simulink model "gyroscope_test"  (R2019a)
settings: Solver=FixedStepAuto  StartTime=0.0  StopTime=30  FixedStep=0.001  RelTol=1e-3
undefined symbols (not defined in the file): gyro_noise
libraries: simulink x6, simulink_extras x5, aerolibnav x2
settings Model: Creator=asmialek  LastModifiedBy=asmialek

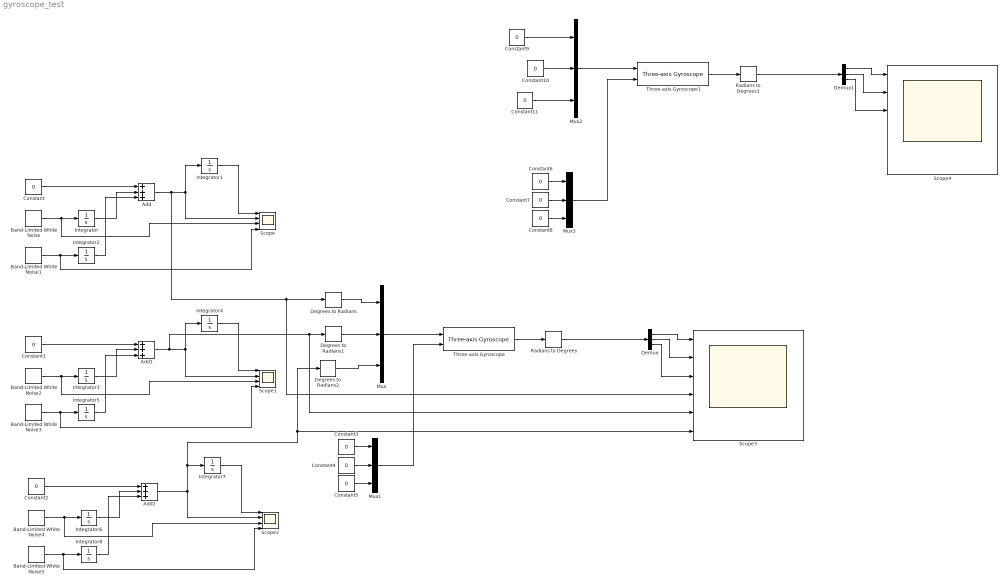
== system gyroscope_test ==
  Add : Sum  Inputs=+++
  Add1 : Sum  Inputs=+++
  Add2 : Sum  Inputs=+++
  Band-Limited White Noise : simulink/Sources/Band-Limited White Noise  Cov=0.002  Ts=10  seed=[233341]
  Band-Limited White Noise1 : simulink/Sources/Band-Limited White Noise  Cov=0.00001  Ts=1  seed=[23341]
  Band-Limited White Noise2 : simulink/Sources/Band-Limited White Noise  Cov=0.002  Ts=10  seed=[233341]
  Band-Limited White Noise3 : simulink/Sources/Band-Limited White Noise  Cov=0.00001  Ts=1  seed=[23341]
  Band-Limited White Noise4 : simulink/Sources/Band-Limited White Noise  Cov=0.002  Ts=10  seed=[233341]
  Band-Limited White Noise5 : simulink/Sources/Band-Limited White Noise  Cov=0.00001  Ts=1  seed=[23341]
  Constant{,1..11} (12 alike) : Constant  Value=0
  Degrees to Radians : simulink_extras/Transformations/Degrees to Radians
  Degrees to Radians1 : simulink_extras/Transformations/Degrees to Radians
  Degrees to Radians2 : simulink_extras/Transformations/Degrees to Radians
  Demux : Demux  Outputs=3
  Demux1 : Demux  Outputs=3
  Integrator{,1..8} (9 alike) : Integrator
  Mux{,1..3} (4 alike) : Mux  Inputs=3
  Radians to Degrees : simulink_extras/Transformations/Radians to Degrees
  Radians to Degrees1 : simulink_extras/Transformations/Radians to Degrees
  Scope : Scope  NumInputPorts=4
  Scope1 : Scope  NumInputPorts=4
  Scope2 : Scope  NumInputPorts=4
  Scope3 : Scope  NumInputPorts=6
  Scope4 : Scope  NumInputPorts=6
  Three-axis Gyroscope : aerolibnav/Three-axis Gyroscope  dtype_g=on  w_g=1  z_g=0  g_sf_cc=[1 0 0; 0 1 0; 0 0 1]  g_bias=[0 0 0]  g_sen=[0 0 0]  g_Ts=0  g_rand=on  g_seeds=[23093 23094 23095]  g_pow=[gyro_noise gyro_noise gyro_noise]  g_sat="[-inf  -inf  -inf  inf inf inf]"
      settings: SourceProductName=Aerospace Blockset  SourceProductBaseCode=AE
  Three-axis Gyroscope1 : aerolibnav/Three-axis Gyroscope  dtype_g=off  w_g=1  z_g=0  g_sf_cc=[1 0 0; 0 1 0; 0 0 1]  g_bias=[0 0 0]  g_sen=[0 0 0]  g_Ts=0.01  g_rand=on  g_seeds=[23093 23094 23095]  g_pow=[gyro_noise gyro_noise gyro_noise]  g_sat="[-inf  -inf  -inf  inf inf inf]"
      settings: SourceProductName=Aerospace Blockset  SourceProductBaseCode=AE
  wires:
  Band-Limited White Noise/1 -> Scope/3, Integrator/1
  Integrator/1 -> Add/2
  Constant/1 -> Add/1
  Add/1 -> Scope3/4, Degrees to Radians/1, Integrator1/1, Scope/2
  Integrator2/1 -> Add/3
  Band-Limited White Noise1/1 -> Scope/4, Integrator2/1
  Integrator1/1 -> Scope/1
  Band-Limited White Noise2/1 -> Scope1/3, Integrator3/1
  Constant1/1 -> Add1/1
  Add1/1 -> Scope3/5, Degrees to Radians1/1, Integrator4/1, Scope1/2
  Integrator3/1 -> Add1/2
  Integrator4/1 -> Scope1/1
  Band-Limited White Noise3/1 -> Scope1/4, Integrator5/1
  Integrator5/1 -> Add1/3
  Band-Limited White Noise4/1 -> Scope2/3, Integrator6/1
  Constant2/1 -> Add2/1
  Add2/1 -> Degrees to Radians2/1, Scope3/6, Integrator7/1, Scope2/2
  Integrator6/1 -> Add2/2
  Integrator7/1 -> Scope2/1
  Band-Limited White Noise5/1 -> Scope2/4, Integrator8/1
  Integrator8/1 -> Add2/3
  Degrees to Radians/1 -> Mux/1
  Degrees to Radians1/1 -> Mux/2
  Degrees to Radians2/1 -> Mux/3
  Mux/1 -> Three-axis Gyroscope/1
  Demux/1 -> Scope3/1
  Demux/2 -> Scope3/2
  Demux/3 -> Scope3/3
  Three-axis Gyroscope/1 -> Radians to Degrees/1
  Constant4/1 -> Mux1/2
  Constant3/1 -> Mux1/1
  Constant5/1 -> Mux1/3
  Mux1/1 -> Three-axis Gyroscope/2
  Radians to Degrees/1 -> Demux/1
  Mux2/1 -> Three-axis Gyroscope1/1
  Constant8/1 -> Mux3/3
  Demux1/1 -> Scope4/1
  Three-axis Gyroscope1/1 -> Radians to Degrees1/1
  Demux1/3 -> Scope4/3
  Constant7/1 -> Mux3/2
  Demux1/2 -> Scope4/2
  Constant6/1 -> Mux3/1
  Mux3/1 -> Three-axis Gyroscope1/2
  Radians to Degrees1/1 -> Demux1/1
  Constant9/1 -> Mux2/1
  Constant11/1 -> Mux2/3
  Constant10/1 -> Mux2/2
